simulink model "VanDerPolSimulink"  (R2024b)
settings: Solver=VariableStepAuto  StartTime=0.0  StopTime=30.0  RelTol=1e-3
values from neighbouring files (symbols this model uses):
  a = 0.5    [VanDerPolScript.m]
  p = [0, 1]    [VanDerPolScript.m]
settings Model: Creator=lukiq  LastModifiedBy=lukiq

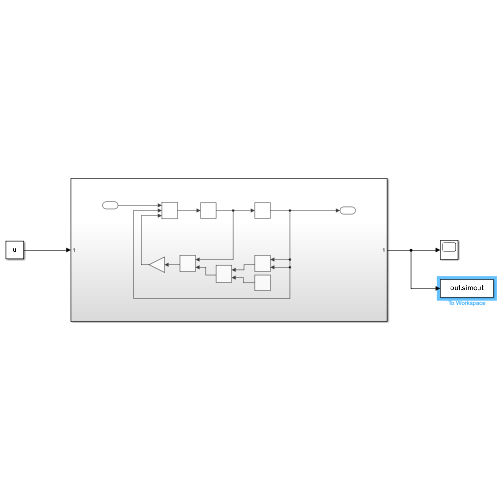
[thumbnail: Simulink's stored preview of the top-level diagram]
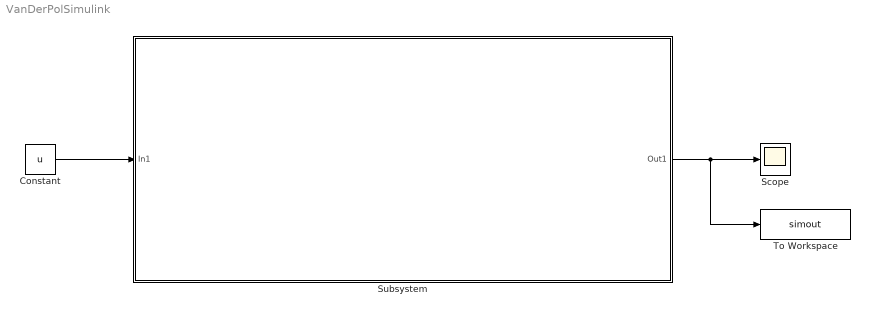
== system VanDerPolSimulink ==
  Constant : Constant  Value=u
  Scope : Scope
  Subsystem : Subsystem
  To Workspace : ToWorkspace  VariableName=simout  SaveFormat=Timeseries  SampleTime=-1
  wires:
  Constant/1 -> Subsystem/1(In1)
  Subsystem/1(Out1) -> To Workspace/1, Scope/1

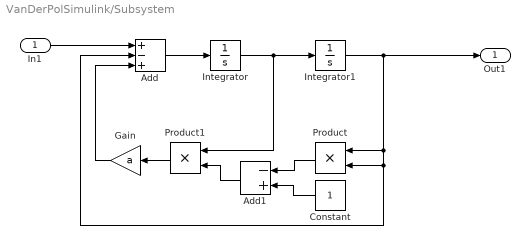
== system VanDerPolSimulink/Subsystem ==
  In1 : Inport
  Add : Sum  Inputs=+-+
  Add1 : Sum  Inputs=-+
  Constant : Constant
  Gain : Gain  Gain=a
  Integrator : Integrator  InitialCondition=p(2)
  Integrator1 : Integrator  InitialCondition=p(1)
  Product : Product
  Product1 : Product
  Out1 : Outport
  wires:
  In1/1 -> Add/1
  Add/1 -> Integrator/1
  Constant/1 -> Add1/2
  Integrator/1 -> Product1/1, Integrator1/1
  Integrator1/1 -> Out1/1, Add/2, Product/2, Product/1
  Product/1 -> Add1/1
  Product1/1 -> Gain/1
  Add1/1 -> Product1/2
  Gain/1 -> Add/3
